simulink library "mech_flyball_lib"  (Simulink 6.0)
settings: Solver=ode45  SolverMode=SingleTasking  StartTime=0.0  StopTime=10.0  RelTol=1e-3
undefined symbols (not defined in the file or in its folder): mech_flyball_rod_inertia, mech_flyball_rod_mass
libraries: mblibv1 x6
settings Model: Creator=nbrewton  LastModifiedBy=batserve  ExtModeAutoUpdateStatusClock=off
settings OptimizationCC: BooleanDataType=off
settings DebuggingCC: SolverPrmCheckMsg=none
settings HardwareCC: TargetUnknown=on

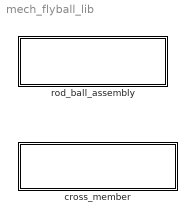
== system mech_flyball_lib ==
  cross_member : Subsystem  mask{rod_length=0, rod_radius=0, density=0}
      mask prompts: rod_length "Length (cm)"; rod_radius "Radius (cm)"; density "Denisty (g/cm^3)"
  rod_ball_assembly : Subsystem  Orientation=left  mask{ball_radius=0, rod_radius=1, rod_length=1, hookup_length=1, density=1, rotation=0}
      mask prompts: ball_radius "Radius of Ball (cm)"; rod_radius "Radius of Rod (cm)"; rod_length "Length of rod (cm)"; hookup_length "Hookup Length (cm)"; density "Material Density (g/cm^3)"; rotation "Rotation (rad)"

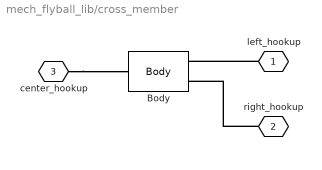
== system mech_flyball_lib/cross_member ==
  Body : mblibv1/Bodies/Body  PhysicalDomain=mechanical  SubClassName=Unknown  PortType=workingframe  LConnTagsString=CG  RConnTagsString=CS1|CS2  DialogClass=MechanicalBodyBlock  Mass=mech_flyball_rod_mass(rod_length, rod_radius, density)  MassUnits=g  InertiaUnits=g*cm^2  Inertia=mech_flyball_rod_inertia(rod_length, rod_radius, density, [1 0 0])  Shape=Cylinder  ShapeDims=[1 1]  ShapeUnits=m  ShapeUse=false  Density=1  DensityUnits=kg/m^3  DensityUse=false  CG=Left$CG$[0 0 0]$ADJOINING$ADJOINING$cm$[0 0 0]$Euler X-Y-Z$deg$WORLD$true  WorkingFrames=Right$CS1$-[rod_length 0 0]/2$CG$CG$cm$[0 0 0]$Euler X-Y-Z$deg$WORLD$true#Right$CS2$[rod_length 0 0]/2$CG$CG$cm$[0 0 0]$Euler X-Y-Z$deg$WORLD$true
  left_hookup : PMIOPort  Orientation=left  Port=1  Side=Left
  right_hookup : PMIOPort  Orientation=left  Port=2  Side=Left
  center_hookup : PMIOPort  Port=3  Side=Right
  connections:
  left_hookup/RConn1 -- Body/RConn1
  right_hookup/RConn1 -- Body/RConn2
  center_hookup/RConn1 -- Body/LConn1

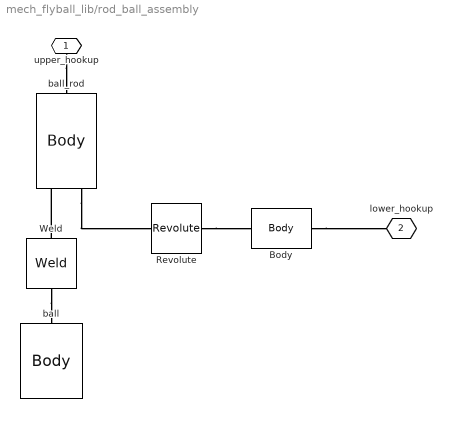
== system mech_flyball_lib/rod_ball_assembly ==
  Body : mblibv1/Bodies/Body  PhysicalDomain=mechanical  SubClassName=Unknown  PortType=workingframe  LConnTagsString=CS1  RConnTagsString=CS2  DialogClass=MechanicalBodyBlock  Mass=mech_flyball_rod_mass(hookup_length, rod_radius, density)  MassUnits=g  InertiaUnits=g*cm^2  Inertia=mech_flyball_rod_inertia(hookup_length, rod_radius, density, [0 0 1])  Shape=Cylinder  ShapeDims=[1 1]  ShapeUnits=m  ShapeUse=false  Density=1  DensityUnits=kg/m^3  DensityUse=false  CG=Left$CG$-[0 0 hookup_length]/2$CS1$CS1$cm$[0 0 0]$Euler X-Y-Z$rad$CS1$false  WorkingFrames=Left$CS1$[0 0 0]$ADJOINING$ADJOINING$cm$[0 -2*rotation 0]$Euler X-Y-Z$rad$ADJOINING$true#Right$CS2$-[0 0 hookup_length]$CS1$CS1$cm$[0 0 0]$Euler X-Y-Z$rad$CS1$true
  Revolute : mblibv1/Joints/Revolute  PhysicalDomain=mechanical  SubClassName=Unknown  PortType=blob  LConnTagsString=__newl0  RConnTagsString=__newr0  NumSAPorts=0  CutJoint=off  MarkAsCut=off  Primitives=revolute  PrimitiveProps=R1$WORLD$[0 1 0]$revolute  DialogClass=JointBlock
  Weld : mblibv1/Joints/Weld  Orientation=down  PhysicalDomain=mechanical  SubClassName=Unknown  PortType=blob  LConnTagsString=__newl0  RConnTagsString=__newr0  NumSAPorts=0  CutJoint=off  MarkAsCut=off  Primitives=weld  PrimitiveProps=W$INERTIAL$[0 0 0]$weld  DialogClass=JointBlock
  ball : mblibv1/Bodies/Body  Orientation=down  PhysicalDomain=mechanical  SubClassName=Unknown  PortType=workingframe  LConnTagsString=CS1  DialogClass=MechanicalBodyBlock  Mass=(density*4*pi*ball_radius^3)/3  MassUnits=g  InertiaUnits=g*cm^2  Inertia=eye(3)*2*(density*4*pi*ball_radius^3)/(3*5)*ball_radius^2  Shape=Cylinder  ShapeDims=[1 1]  ShapeUnits=m  ShapeUse=false  Density=1  DensityUnits=kg/m^3  DensityUse=false  CG=Left$CG$-[0 0 ball_radius]$CS1$CS1$cm$[0 0 0]$Euler X-Y-Z$deg$CS1$false  WorkingFrames=Left$CS1$[0 0 0]$ADJOINING$ADJOINING$cm$[0 0 0]$Euler X-Y-Z$deg$ADJOINING$true
  ball_rod : mblibv1/Bodies/Body  Orientation=down  PhysicalDomain=mechanical  SubClassName=Unknown  PortType=workingframe  LConnTagsString=CS1  RConnTagsString=CS2|CS3  DialogClass=MechanicalBodyBlock  Mass=mech_flyball_rod_mass(rod_length, rod_radius, density)  MassUnits=g  InertiaUnits=g*cm^2  Inertia=mech_flyball_rod_inertia(rod_length, rod_radius, density, [0 0 1])  Shape=Cylinder  ShapeDims=[1 1]  ShapeUnits=m  ShapeUse=false  Density=1  DensityUnits=kg/m^3  DensityUse=false  CG=Left$CG$-[0 0 rod_length]/2$CS1$CS1$cm$[0 0 0]$Euler X-Y-Z$rad$CS1$false  WorkingFrames=Left$CS1$[0 0 0]$ADJOINING$ADJOINING$cm$[0 rotation 0]$Euler X-Y-Z$rad$ADJOINING$true#Right$CS2$-[0 0 rod_length]$CS1$CS1$cm$[0 0 0]$Euler X-Y-Z$rad$CS1$true#Right$CS3$-[0 0 hookup_length]$CS1$CS1$cm$[0 0 0]$Euler X-Y-Z$rad$CS1$true
  upper_hookup : PMIOPort  Orientation=down  Port=1  Side=Right
  lower_hookup : PMIOPort  Orientation=left  Port=2  Side=Left
  connections:
  upper_hookup/RConn1 -- ball_rod/LConn1
  Weld/LConn1 -- ball_rod/RConn1
  Weld/RConn1 -- ball/LConn1
  Body/RConn1 -- lower_hookup/RConn1
  ball_rod/RConn2 -- Revolute/LConn1
  Revolute/RConn1 -- Body/LConn1
